simulink model "case1"  (R2024b)
settings: Solver=FixedStepAuto  StartTime=0  StopTime=1  FixedStep=1e-7  RelTol=1e-3
values from neighbouring files (symbols this model uses):
  SG_D_1_D = 0.01056    [IEEE9_case_parameters.m]    (also in case1_parameters.m; case2_parameters.m; case3_parameters.m; case4_parameters.m)
  SG_D_1_EnableSaturation = 0    [IEEE9_case_parameters.m]    (also in case1_parameters.m; case2_parameters.m; case3_parameters.m; case4_parameters.m)
  SG_D_1_f0 = 60    [IEEE9_case_parameters.m]    (also in case1_parameters.m; case2_parameters.m; case3_parameters.m; case4_parameters.m)
  SG_D_1_H = 7.5    [IEEE9_case_parameters.m]    (also in case1_parameters.m; case2_parameters.m; case3_parameters.m; case4_parameters.m)
  SG_D_1_K_A = 20    [IEEE9_case_parameters.m]    (also in case1_parameters.m; case2_parameters.m; case3_parameters.m; case4_parameters.m)
  SG_D_1_K_E = 1.000000e+1    (= 10)    [IEEE9_case_parameters.m]    (also in case1_parameters.m; case2_parameters.m; case3_parameters.m; case4_parameters.m)
  SG_D_1_K_F = 2.363    [IEEE9_case_parameters.m]    (also in case1_parameters.m; case2_parameters.m; case3_parameters.m; case4_parameters.m)
  SG_D_1_K_s = 0.5    [IEEE9_case_parameters.m]    (also in case1_parameters.m = 5; case2_parameters.m = 5; case3_parameters.m = 5; case4_parameters.m = 5)
  SG_D_1_R_a = 0.001088    [IEEE9_case_parameters.m]    (also in case1_parameters.m; case2_parameters.m; case3_parameters.m; case4_parameters.m)
  SG_D_1_S_A = 1    [IEEE9_case_parameters.m]    (also in case1_parameters.m; case2_parameters.m; case3_parameters.m; case4_parameters.m)
  SG_D_1_S_B = 0.103    [IEEE9_case_parameters.m]    (also in case1_parameters.m; case2_parameters.m; case3_parameters.m; case4_parameters.m)
  SG_D_1_S_N = 10.659857    [IEEE9_case_parameters.m]    (also in case1_parameters.m; case2_parameters.m; case3_parameters.m; case4_parameters.m)
  SG_D_1_SpeedPara = 200    [IEEE9_case_parameters.m]    (also in case1_parameters.m; case2_parameters.m; case3_parameters.m; case4_parameters.m)
  SG_D_1_T_0 = 0.720173    [IEEE9_case_parameters.m]    (also in case1_parameters.m = 0.755522; case2_parameters.m = 0.808931; case3_parameters.m = 0.869402; case4_parameters.m = 0.729316)
  SG_D_1_T_1 = 0.3    [IEEE9_case_parameters.m]    (also in case1_parameters.m; case2_parameters.m; case3_parameters.m; case4_parameters.m)
  SG_D_1_T_2 = 0.05    [IEEE9_case_parameters.m]    (also in case1_parameters.m; case2_parameters.m; case3_parameters.m; case4_parameters.m)
  SG_D_1_T_3 = 0.02    [IEEE9_case_parameters.m]    (also in case1_parameters.m; case2_parameters.m; case3_parameters.m; case4_parameters.m)
  SG_D_1_T_4 = 0.005    [IEEE9_case_parameters.m]    (also in case1_parameters.m; case2_parameters.m; case3_parameters.m; case4_parameters.m)
  SG_D_1_T_A = 0.02    [IEEE9_case_parameters.m]    (also in case1_parameters.m; case2_parameters.m; case3_parameters.m; case4_parameters.m)
  SG_D_1_T_dd = 8.000000e+0    (= 8)    [IEEE9_case_parameters.m]    (also in case1_parameters.m; case2_parameters.m; case3_parameters.m; case4_parameters.m)
  SG_D_1_T_ddd = 0.04    [IEEE9_case_parameters.m]    (also in case1_parameters.m; case2_parameters.m; case3_parameters.m; case4_parameters.m)
  SG_D_1_T_E = 0.314    [IEEE9_case_parameters.m]    (also in case1_parameters.m; case2_parameters.m; case3_parameters.m; case4_parameters.m)
  SG_D_1_T_F = 0.35    [IEEE9_case_parameters.m]    (also in case1_parameters.m; case2_parameters.m; case3_parameters.m; case4_parameters.m)
  SG_D_1_T_qd = 0.8    [IEEE9_case_parameters.m]    (also in case1_parameters.m; case2_parameters.m; case3_parameters.m; case4_parameters.m)
  SG_D_1_T_qdd = 0.02    [IEEE9_case_parameters.m]    (also in case1_parameters.m; case2_parameters.m; case3_parameters.m; case4_parameters.m)
  SG_D_1_T_speed = 0.1    [IEEE9_case_parameters.m]    (also in case1_parameters.m = 200; case2_parameters.m = 200; case3_parameters.m = 200; case4_parameters.m = 200)
  SG_D_1_T_w = 0.5    [IEEE9_case_parameters.m]    (also in case1_parameters.m; case2_parameters.m; case3_parameters.m; case4_parameters.m)
  SG_D_1_V_ref = 1.990276    [IEEE9_case_parameters.m]    (also in case1_parameters.m = 2.042296; case2_parameters.m = 2.051388; case3_parameters.m = 2.089584; case4_parameters.m = 2.01845)
  SG_D_1_w_ref = 376.991118    [IEEE9_case_parameters.m]    (also in case1_parameters.m; case2_parameters.m; case3_parameters.m; case4_parameters.m)
  SG_D_1_wb = 6.000000e+1    (= 60)    [IEEE9_case_parameters.m]    (also in case1_parameters.m; case2_parameters.m; case3_parameters.m; case4_parameters.m)
  SG_D_1_x_d = 1.9    [IEEE9_case_parameters.m]    (also in case1_parameters.m; case2_parameters.m; case3_parameters.m; case4_parameters.m)
  SG_D_1_x_dd = 0.302    [IEEE9_case_parameters.m]    (also in case1_parameters.m; case2_parameters.m; case3_parameters.m; case4_parameters.m)
  SG_D_1_x_ddd = 0.204    [IEEE9_case_parameters.m]    (also in case1_parameters.m; case2_parameters.m; case3_parameters.m; case4_parameters.m)
  SG_D_1_x_l = 0.05    [IEEE9_case_parameters.m]    (also in case1_parameters.m; case2_parameters.m; case3_parameters.m; case4_parameters.m)
  SG_D_1_x_q = 1.3    [IEEE9_case_parameters.m]    (also in case1_parameters.m; case2_parameters.m; case3_parameters.m; case4_parameters.m)
  SG_D_1_x_qd = 0.5    [IEEE9_case_parameters.m]    (also in case1_parameters.m; case2_parameters.m; case3_parameters.m; case4_parameters.m)
  SG_D_1_x_qdd = 0.3    [IEEE9_case_parameters.m]    (also in case1_parameters.m; case2_parameters.m; case3_parameters.m; case4_parameters.m)
  SG_D_2_D = 0.02    [IEEE9_case_parameters.m]    (also in case1_parameters.m; case2_parameters.m; case3_parameters.m; case4_parameters.m)
  SG_D_2_EnableSaturation = 0    [IEEE9_case_parameters.m]    (also in case1_parameters.m; case2_parameters.m; case3_parameters.m; case4_parameters.m)
  SG_D_2_f0 = 60    [IEEE9_case_parameters.m]    (also in case1_parameters.m; case2_parameters.m; case3_parameters.m; case4_parameters.m)
  SG_D_2_H = 8.000000e+0    (= 8)    [IEEE9_case_parameters.m]    (also in case1_parameters.m; case2_parameters.m; case3_parameters.m; case4_parameters.m)
  SG_D_2_K_A = 20    [IEEE9_case_parameters.m]    (also in case1_parameters.m; case2_parameters.m; case3_parameters.m; case4_parameters.m)
  SG_D_2_K_E = 1.000000e+1    (= 10)    [IEEE9_case_parameters.m]    (also in case1_parameters.m; case2_parameters.m; case3_parameters.m; case4_parameters.m)
  SG_D_2_K_F = 2.363    [IEEE9_case_parameters.m]    (also in case1_parameters.m; case2_parameters.m; case3_parameters.m; case4_parameters.m)
  SG_D_2_K_s = 0.5    [IEEE9_case_parameters.m]    (also in case1_parameters.m = 4; case2_parameters.m = 4; case3_parameters.m = 4; case4_parameters.m = 4)
  SG_D_2_R_a = 0.001088    [IEEE9_case_parameters.m]    (also in case1_parameters.m; case2_parameters.m; case3_parameters.m; case4_parameters.m)
  SG_D_2_S_A = 1    [IEEE9_case_parameters.m]    (also in case1_parameters.m; case2_parameters.m; case3_parameters.m; case4_parameters.m)
  SG_D_2_S_B = 0.103    [IEEE9_case_parameters.m]    (also in case1_parameters.m; case2_parameters.m; case3_parameters.m; case4_parameters.m)
  SG_D_2_S_N = 10.659857    [IEEE9_case_parameters.m]    (also in case1_parameters.m; case2_parameters.m; case3_parameters.m; case4_parameters.m)
  SG_D_2_SpeedPara = 200    [IEEE9_case_parameters.m]    (also in case1_parameters.m; case2_parameters.m; case3_parameters.m; case4_parameters.m)
  SG_D_2_T_0 = 1.632913    [IEEE9_case_parameters.m]    (also in case1_parameters.m = 1.632925; case2_parameters.m = 1.632915; case3_parameters.m = 1.632914; case4_parameters.m = 1.632927)
  SG_D_2_T_1 = 0.2    [IEEE9_case_parameters.m]    (also in case1_parameters.m; case2_parameters.m; case3_parameters.m; case4_parameters.m)
  SG_D_2_T_2 = 0.05    [IEEE9_case_parameters.m]    (also in case1_parameters.m; case2_parameters.m; case3_parameters.m; case4_parameters.m)
  SG_D_2_T_3 = 0.02    [IEEE9_case_parameters.m]    (also in case1_parameters.m; case2_parameters.m; case3_parameters.m; case4_parameters.m)
  SG_D_2_T_4 = 0.005    [IEEE9_case_parameters.m]    (also in case1_parameters.m; case2_parameters.m; case3_parameters.m; case4_parameters.m)
  SG_D_2_T_A = 0.02    [IEEE9_case_parameters.m]    (also in case1_parameters.m; case2_parameters.m; case3_parameters.m; case4_parameters.m)
  SG_D_2_T_dd = 7.9    [IEEE9_case_parameters.m]    (also in case1_parameters.m; case2_parameters.m; case3_parameters.m; case4_parameters.m)
  SG_D_2_T_ddd = 0.04    [IEEE9_case_parameters.m]    (also in case1_parameters.m; case2_parameters.m; case3_parameters.m; case4_parameters.m)
  SG_D_2_T_E = 0.314    [IEEE9_case_parameters.m]    (also in case1_parameters.m; case2_parameters.m; case3_parameters.m; case4_parameters.m)
  SG_D_2_T_F = 0.35    [IEEE9_case_parameters.m]    (also in case1_parameters.m; case2_parameters.m; case3_parameters.m; case4_parameters.m)
  SG_D_2_T_qd = 0.8    [IEEE9_case_parameters.m]    (also in case1_parameters.m; case2_parameters.m; case3_parameters.m; case4_parameters.m)
  SG_D_2_T_qdd = 0.015    [IEEE9_case_parameters.m]    (also in case1_parameters.m; case2_parameters.m; case3_parameters.m; case4_parameters.m)
  SG_D_2_T_speed = 0.1    [IEEE9_case_parameters.m]    (also in case1_parameters.m = 150; case2_parameters.m = 150; case3_parameters.m = 150; case4_parameters.m = 150)
  SG_D_2_T_w = 0.35    [IEEE9_case_parameters.m]    (also in case1_parameters.m; case2_parameters.m; case3_parameters.m; case4_parameters.m)
  SG_D_2_V_ref = 2.58547    [IEEE9_case_parameters.m]    (also in case1_parameters.m = 2.597896; case2_parameters.m = 2.587136; case3_parameters.m = 2.586042; case4_parameters.m = 2.599679)
  SG_D_2_w_ref = 376.991118    [IEEE9_case_parameters.m]    (also in case1_parameters.m; case2_parameters.m; case3_parameters.m; case4_parameters.m)
  SG_D_2_wb = 6.000000e+1    (= 60)    [IEEE9_case_parameters.m]    (also in case1_parameters.m; case2_parameters.m; case3_parameters.m; case4_parameters.m)
  SG_D_2_x_d = 1.8    [IEEE9_case_parameters.m]    (also in case1_parameters.m; case2_parameters.m; case3_parameters.m; case4_parameters.m)
  SG_D_2_x_dd = 0.302    [IEEE9_case_parameters.m]    (also in case1_parameters.m; case2_parameters.m; case3_parameters.m; case4_parameters.m)
  SG_D_2_x_ddd = 0.204    [IEEE9_case_parameters.m]    (also in case1_parameters.m; case2_parameters.m; case3_parameters.m; case4_parameters.m)
  SG_D_2_x_l = 0.05    [IEEE9_case_parameters.m]    (also in case1_parameters.m; case2_parameters.m; case3_parameters.m; case4_parameters.m)
  SG_D_2_x_q = 1.25    [IEEE9_case_parameters.m]    (also in case1_parameters.m; case2_parameters.m; case3_parameters.m; case4_parameters.m)
  SG_D_2_x_qd = 0.5    [IEEE9_case_parameters.m]    (also in case1_parameters.m; case2_parameters.m; case3_parameters.m; case4_parameters.m)
  SG_D_2_x_qdd = 0.3    [IEEE9_case_parameters.m]    (also in case1_parameters.m; case2_parameters.m; case3_parameters.m; case4_parameters.m)
  SG_D_3_D = 0.02    [IEEE9_case_parameters.m]    (also in case1_parameters.m; case2_parameters.m; case3_parameters.m; case4_parameters.m)
  SG_D_3_EnableSaturation = 0    [IEEE9_case_parameters.m]    (also in case1_parameters.m; case2_parameters.m; case3_parameters.m; case4_parameters.m)
  SG_D_3_f0 = 60    [IEEE9_case_parameters.m]    (also in case1_parameters.m; case2_parameters.m; case3_parameters.m; case4_parameters.m)
  SG_D_3_H = 7.7    [IEEE9_case_parameters.m]    (also in case1_parameters.m; case2_parameters.m; case3_parameters.m; case4_parameters.m)
  SG_D_3_K_A = 20    [IEEE9_case_parameters.m]    (also in case1_parameters.m; case2_parameters.m; case3_parameters.m; case4_parameters.m)
  SG_D_3_K_E = 1.000000e+1    (= 10)    [IEEE9_case_parameters.m]    (also in case1_parameters.m; case2_parameters.m; case3_parameters.m; case4_parameters.m)
  SG_D_3_K_F = 2.363    [IEEE9_case_parameters.m]    (also in case1_parameters.m; case2_parameters.m; case3_parameters.m; case4_parameters.m)
  SG_D_3_K_s = 0.2    [IEEE9_case_parameters.m]    (also in case1_parameters.m = 2; case2_parameters.m = 2; case3_parameters.m = 2; case4_parameters.m = 2)
  SG_D_3_R_a = 0.001088    [IEEE9_case_parameters.m]    (also in case1_parameters.m; case2_parameters.m; case3_parameters.m; case4_parameters.m)
  SG_D_3_S_A = 1    [IEEE9_case_parameters.m]    (also in case1_parameters.m; case2_parameters.m; case3_parameters.m; case4_parameters.m)
  SG_D_3_S_B = 0.103    [IEEE9_case_parameters.m]    (also in case1_parameters.m; case2_parameters.m; case3_parameters.m; case4_parameters.m)
  SG_D_3_S_N = 10.659857    [IEEE9_case_parameters.m]    (also in case1_parameters.m; case2_parameters.m; case3_parameters.m; case4_parameters.m)
  SG_D_3_SpeedPara = 200    [IEEE9_case_parameters.m]    (also in case1_parameters.m; case2_parameters.m; case3_parameters.m; case4_parameters.m)
  SG_D_3_T_0 = 0.850788    [IEEE9_case_parameters.m]    (also in case1_parameters.m = 0.850786; case2_parameters.m = 0.850787; case3_parameters.m; case4_parameters.m = 0.850786)
  SG_D_3_T_1 = 0.2    [IEEE9_case_parameters.m]    (also in case1_parameters.m; case2_parameters.m; case3_parameters.m; case4_parameters.m)
  SG_D_3_T_2 = 0.05    [IEEE9_case_parameters.m]    (also in case1_parameters.m; case2_parameters.m; case3_parameters.m; case4_parameters.m)
  SG_D_3_T_3 = 0.02    [IEEE9_case_parameters.m]    (also in case1_parameters.m; case2_parameters.m; case3_parameters.m; case4_parameters.m)
  SG_D_3_T_4 = 0.005    [IEEE9_case_parameters.m]    (also in case1_parameters.m; case2_parameters.m; case3_parameters.m; case4_parameters.m)
  SG_D_3_T_A = 0.02    [IEEE9_case_parameters.m]    (also in case1_parameters.m; case2_parameters.m; case3_parameters.m; case4_parameters.m)
  SG_D_3_T_dd = 8.1    [IEEE9_case_parameters.m]    (also in case1_parameters.m; case2_parameters.m; case3_parameters.m; case4_parameters.m)
  SG_D_3_T_ddd = 0.04    [IEEE9_case_parameters.m]    (also in case1_parameters.m; case2_parameters.m; case3_parameters.m; case4_parameters.m)
  SG_D_3_T_E = 0.314    [IEEE9_case_parameters.m]    (also in case1_parameters.m; case2_parameters.m; case3_parameters.m; case4_parameters.m)
  SG_D_3_T_F = 0.35    [IEEE9_case_parameters.m]    (also in case1_parameters.m; case2_parameters.m; case3_parameters.m; case4_parameters.m)
  SG_D_3_T_qd = 0.8    [IEEE9_case_parameters.m]    (also in case1_parameters.m; case2_parameters.m; case3_parameters.m; case4_parameters.m)
  SG_D_3_T_qdd = 0.015    [IEEE9_case_parameters.m]    (also in case1_parameters.m; case2_parameters.m; case3_parameters.m; case4_parameters.m)
  SG_D_3_T_speed = 0.1    [IEEE9_case_parameters.m]    (also in case1_parameters.m = 180; case2_parameters.m = 180; case3_parameters.m = 180; case4_parameters.m = 180)
  SG_D_3_T_w = 0.4    [IEEE9_case_parameters.m]    (also in case1_parameters.m; case2_parameters.m; case3_parameters.m; case4_parameters.m)
  SG_D_3_V_ref = 1.892727    [IEEE9_case_parameters.m]    (also in case1_parameters.m = 1.906439; case2_parameters.m = 1.895535; case3_parameters.m = 1.892105; case4_parameters.m = 1.906598)
  SG_D_3_w_ref = 376.991118    [IEEE9_case_parameters.m]    (also in case1_parameters.m; case2_parameters.m; case3_parameters.m; case4_parameters.m)
  SG_D_3_wb = 6.000000e+1    (= 60)    [IEEE9_case_parameters.m]    (also in case1_parameters.m; case2_parameters.m; case3_parameters.m; case4_parameters.m)
  SG_D_3_x_d = 1.85    [IEEE9_case_parameters.m]    (also in case1_parameters.m; case2_parameters.m; case3_parameters.m; case4_parameters.m)
  SG_D_3_x_dd = 0.302    [IEEE9_case_parameters.m]    (also in case1_parameters.m; case2_parameters.m; case3_parameters.m; case4_parameters.m)
  SG_D_3_x_ddd = 0.204    [IEEE9_case_parameters.m]    (also in case1_parameters.m; case2_parameters.m; case3_parameters.m; case4_parameters.m)
  SG_D_3_x_l = 0.05    [IEEE9_case_parameters.m]    (also in case1_parameters.m; case2_parameters.m; case3_parameters.m; case4_parameters.m)
  SG_D_3_x_q = 1.2    [IEEE9_case_parameters.m]    (also in case1_parameters.m; case2_parameters.m; case3_parameters.m; case4_parameters.m)
  SG_D_3_x_qd = 0.5    [IEEE9_case_parameters.m]    (also in case1_parameters.m; case2_parameters.m; case3_parameters.m; case4_parameters.m)
  SG_D_3_x_qdd = 0.3    [IEEE9_case_parameters.m]    (also in case1_parameters.m; case2_parameters.m; case3_parameters.m; case4_parameters.m)
(part 3 of 12)

== system case1/AC_1/d_id_load_7_block ==
  note: d_id_load_7 in case1
      | $376.991118430775\,\mathrm{iq}_{\mathrm{load},7}-1025.52197474754\,\mathrm{id}_{\mathrm{load},7}+1219.07936641917\,\mathrm{vd}_{\mathrm{bus},7}$
      | Automatically generated on 2025-10-31 18:50:38 .
  State_id_load_7_7e244 : Inport
  State_iq_load_7_7baed : Inport  Port=2
  State_vd_bus_7_6ff07 : Inport  Port=3
  Add_61909 : Sum
  Add_b6594 : Sum
  Constant_-1025.52197474754_80390 : Constant  Value=-1025.52197474754
  Constant_1219.07936641917_674e5 : Constant  Value=1219.07936641917
  Constant_376.991118430775_4e2b0 : Constant  Value=376.991118430775
  Product_12f11 : Product
  Product_491b3 : Product
  Product_d0252 : Product
  Blockout_d_id_load_7_3ab02 : Outport
  wires:
  Constant_-1025.52197474754_80390/1 -> Product_12f11/1
  Product_491b3/1 -> Add_b6594/2
  State_id_load_7_7e244/1 -> Product_12f11/2
  Constant_376.991118430775_4e2b0/1 -> Product_491b3/1
  Product_12f11/1 -> Add_b6594/1
  State_iq_load_7_7baed/1 -> Product_491b3/2
  Constant_1219.07936641917_674e5/1 -> Product_d0252/1
  State_vd_bus_7_6ff07/1 -> Product_d0252/2
  Add_b6594/1 -> Add_61909/1
  Product_d0252/1 -> Add_61909/2
  Add_61909/1 -> Blockout_d_id_load_7_3ab02/1

== system case1/AC_1/d_id_load_9_block ==
  note: d_id_load_9 in case1
      | $376.991118430775\,\mathrm{iq}_{\mathrm{load},9}-897.331727994337\,\mathrm{id}_{\mathrm{load},9}+1471.75490379155\,\mathrm{vd}_{\mathrm{bus},9}$
      | Automatically generated on 2025-10-31 18:50:40 .
  State_id_load_9_6175e : Inport
  State_iq_load_9_2b565 : Inport  Port=2
  State_vd_bus_9_97729 : Inport  Port=3
  Add_41749 : Sum
  Add_a1c56 : Sum
  Constant_-897.331727994337_48efa : Constant  Value=-897.331727994337
  Constant_1471.75490379155_76577 : Constant  Value=1471.75490379155
  Constant_376.991118430775_bbee5 : Constant  Value=376.991118430775
  Product_0f7c0 : Product
  Product_ef85c : Product
  Product_fef82 : Product
  Blockout_d_id_load_9_6afbf : Outport
  wires:
  Constant_-897.331727994337_48efa/1 -> Product_0f7c0/1
  Product_fef82/1 -> Add_a1c56/2
  State_id_load_9_6175e/1 -> Product_0f7c0/2
  Constant_376.991118430775_bbee5/1 -> Product_fef82/1
  Product_0f7c0/1 -> Add_a1c56/1
  State_iq_load_9_2b565/1 -> Product_fef82/2
  Constant_1471.75490379155_76577/1 -> Product_ef85c/1
  State_vd_bus_9_97729/1 -> Product_ef85c/2
  Add_a1c56/1 -> Add_41749/1
  Product_ef85c/1 -> Add_41749/2
  Add_41749/1 -> Blockout_d_id_load_9_6afbf/1

== system case1/AC_1/d_iq_line_1_4_block ==
  note: d_iq_line_1_4 in case1
      | $6387.9543042679\,\mathrm{vq}_{\mathrm{bus},1}-376.991118430775\,\mathrm{id}_{\mathrm{line},1,4}-6387.9543042679\,\mathrm{vq}_{\mathrm{bus},4}$
      | Automatically generated on 2025-10-31 18:50:43 .
  State_id_line_1_4_e2784 : Inport
  State_vq_bus_1_cc1a1 : Inport  Port=2
  State_vq_bus_4_b95c1 : Inport  Port=3
  Add_609df : Sum
  Constant_-376.991118430775_4f7c2 : Constant  Value=-376.991118430775
  Constant_6387.9543042679_077c5 : Constant  Value=6387.9543042679
  Constant_6387.9543042679_526d1 : Constant  Value=6387.9543042679
  Product_10305 : Product
  Product_2fb22 : Product
  Product_4450d : Product
  Subtract_016be : Sum  Inputs=+-
  Blockout_d_iq_line_1_4_78aac : Outport
  wires:
  Constant_-376.991118430775_4f7c2/1 -> Product_10305/1
  Product_2fb22/1 -> Add_609df/2
  State_id_line_1_4_e2784/1 -> Product_10305/2
  Constant_6387.9543042679_526d1/1 -> Product_2fb22/1
  Product_10305/1 -> Add_609df/1
  Subtract_016be/1 -> Blockout_d_iq_line_1_4_78aac/1
  State_vq_bus_1_cc1a1/1 -> Product_2fb22/2
  Constant_6387.9543042679_077c5/1 -> Product_4450d/1
  State_vq_bus_4_b95c1/1 -> Product_4450d/2
  Add_609df/1 -> Subtract_016be/1
  Product_4450d/1 -> Subtract_016be/2

== system case1/AC_1/d_iq_line_3_6_block ==
  note: d_iq_line_3_6 in case1
      | $6278.9448451507\,\mathrm{vq}_{\mathrm{bus},3}-376.991118430775\,\mathrm{id}_{\mathrm{line},3,6}-6278.9448451507\,\mathrm{vq}_{\mathrm{bus},6}$
      | Automatically generated on 2025-10-31 18:50:50 .
  State_id_line_3_6_f913b : Inport
  State_vq_bus_3_5a1c9 : Inport  Port=2
  State_vq_bus_6_03933 : Inport  Port=3
  Add_de142 : Sum
  Constant_-376.991118430775_59102 : Constant  Value=-376.991118430775
  Constant_6278.9448451507_1221b : Constant  Value=6278.9448451507
  Constant_6278.9448451507_5b025 : Constant  Value=6278.9448451507
  Product_669f2 : Product
  Product_75886 : Product
  Product_e6f36 : Product
  Subtract_db1d0 : Sum  Inputs=+-
  Blockout_d_iq_line_3_6_784c0 : Outport
  wires:
  Constant_-376.991118430775_59102/1 -> Product_75886/1
  Product_e6f36/1 -> Add_de142/2
  State_id_line_3_6_f913b/1 -> Product_75886/2
  Constant_6278.9448451507_1221b/1 -> Product_e6f36/1
  Product_75886/1 -> Add_de142/1
  State_vq_bus_3_5a1c9/1 -> Product_e6f36/2
  Constant_6278.9448451507_5b025/1 -> Product_669f2/1
  State_vq_bus_6_03933/1 -> Product_669f2/2
  Add_de142/1 -> Subtract_db1d0/1
  Product_669f2/1 -> Subtract_db1d0/2
  Subtract_db1d0/1 -> Blockout_d_iq_line_3_6_784c0/1

== system case1/AC_1/d_iq_line_4_5_block ==
  note: d_iq_line_4_5 in case1
      | $3999.41486875903\,\mathrm{vq}_{\mathrm{bus},4}-70.7030565753656\,\mathrm{iq}_{\mathrm{line},4,5}-376.991118430775\,\mathrm{id}_{\mathrm{line},4,5}-3999.41486875903\,\mathrm{vq}_{\mathrm{bus},5}$
      | Automatically generated on 2025-10-31 18:50:45 .
  State_id_line_4_5_305b5 : Inport
  State_iq_line_4_5_0a9d2 : Inport  Port=2
  State_vq_bus_4_e89f1 : Inport  Port=3
  State_vq_bus_5_04a69 : Inport  Port=4
  Add_d0e3e : Sum
  Constant_-376.991118430775_c3725 : Constant  Value=-376.991118430775
  Constant_3999.41486875903_a8499 : Constant  Value=3999.41486875903
  Constant_3999.41486875903_f6b00 : Constant  Value=3999.41486875903
  Constant_70.7030565753656_055d7 : Constant  Value=70.7030565753656
  Product_4f6ce : Product
  Product_504af : Product
  Product_52caf : Product
  Product_aa46e : Product
  Subtract_8fbf3 : Sum  Inputs=+-
  Subtract_f2a4b : Sum  Inputs=+-
  Blockout_d_iq_line_4_5_e1e40 : Outport
  wires:
  Constant_-376.991118430775_c3725/1 -> Product_504af/1
  Constant_70.7030565753656_055d7/1 -> Product_aa46e/1
  State_id_line_4_5_305b5/1 -> Product_504af/2
  State_iq_line_4_5_0a9d2/1 -> Product_aa46e/2
  Product_504af/1 -> Subtract_8fbf3/1
  Constant_3999.41486875903_a8499/1 -> Product_52caf/1
  Product_aa46e/1 -> Subtract_8fbf3/2
  State_vq_bus_4_e89f1/1 -> Product_52caf/2
  Subtract_8fbf3/1 -> Add_d0e3e/1
  Product_52caf/1 -> Add_d0e3e/2
  Constant_3999.41486875903_f6b00/1 -> Product_4f6ce/1
  State_vq_bus_5_04a69/1 -> Product_4f6ce/2
  Add_d0e3e/1 -> Subtract_f2a4b/1
  Product_4f6ce/1 -> Subtract_f2a4b/2
  Subtract_f2a4b/1 -> Blockout_d_iq_line_4_5_e1e40/1

== system case1/AC_1/d_iq_line_5_6_block ==
  note: d_iq_line_5_6 in case1
      | $2164.38922309312\,\mathrm{vq}_{\mathrm{bus},5}-87.7794349454712\,\mathrm{iq}_{\mathrm{line},5,6}-376.991118430775\,\mathrm{id}_{\mathrm{line},5,6}-2164.38922309312\,\mathrm{vq}_{\mathrm{bus},6}$
      | Automatically generated on 2025-10-31 18:50:48 .
  State_id_line_5_6_4698d : Inport
  State_iq_line_5_6_e5c27 : Inport  Port=2
  State_vq_bus_5_b22ab : Inport  Port=3
  State_vq_bus_6_bf656 : Inport  Port=4
  Add_a83be : Sum
  Constant_-376.991118430775_4d48f : Constant  Value=-376.991118430775
  Constant_2164.38922309312_70a07 : Constant  Value=2164.38922309312
  Constant_2164.38922309312_f6087 : Constant  Value=2164.38922309312
  Constant_87.7794349454712_08c9f : Constant  Value=87.7794349454712
  Product_0ca73 : Product
  Product_18bd1 : Product
  Product_3d32a : Product
  Product_b60ba : Product
  Subtract_1282d : Sum  Inputs=+-
  Subtract_42846 : Sum  Inputs=+-
  Blockout_d_iq_line_5_6_8d1bb : Outport
  wires:
  Constant_-376.991118430775_4d48f/1 -> Product_3d32a/1
  Constant_87.7794349454712_08c9f/1 -> Product_0ca73/1
  Subtract_1282d/1 -> Blockout_d_iq_line_5_6_8d1bb/1
  State_id_line_5_6_4698d/1 -> Product_3d32a/2
  State_iq_line_5_6_e5c27/1 -> Product_0ca73/2
  Product_3d32a/1 -> Subtract_42846/1
  Constant_2164.38922309312_f6087/1 -> Product_b60ba/1
  Product_0ca73/1 -> Subtract_42846/2
  Product_18bd1/1 -> Subtract_1282d/2
  State_vq_bus_5_b22ab/1 -> Product_b60ba/2
  Subtract_42846/1 -> Add_a83be/1
  Product_b60ba/1 -> Add_a83be/2
  Constant_2164.38922309312_70a07/1 -> Product_18bd1/1
  State_vq_bus_6_bf656/1 -> Product_18bd1/2
  Add_a83be/1 -> Subtract_1282d/1

== system case1/AC_1/d_iq_line_6_7_block ==
  note: d_iq_line_6_7 in case1
      | $3650.2596024388\,\mathrm{vq}_{\mathrm{bus},6}-45.1713972564836\,\mathrm{iq}_{\mathrm{line},6,7}-376.991118430775\,\mathrm{id}_{\mathrm{line},6,7}-3650.2596024388\,\mathrm{vq}_{\mathrm{bus},7}$
      | Automatically generated on 2025-10-31 18:50:52 .
  State_id_line_6_7_d6333 : Inport
  State_iq_line_6_7_6494b : Inport  Port=2
  State_vq_bus_6_af623 : Inport  Port=3
  State_vq_bus_7_386f3 : Inport  Port=4
  Add_1f3e0 : Sum
  Constant_-376.991118430775_f3922 : Constant  Value=-376.991118430775
  Constant_3650.2596024388_32c77 : Constant  Value=3650.2596024388
  Constant_3650.2596024388_bb62a : Constant  Value=3650.2596024388
  Constant_45.1713972564836_4ebf7 : Constant  Value=45.1713972564836
  Product_58448 : Product
  Product_5c0e6 : Product
  Product_7400f : Product
  Product_cdcfd : Product
  Subtract_13a48 : Sum  Inputs=+-
  Subtract_ef767 : Sum  Inputs=+-
  Blockout_d_iq_line_6_7_6cbac : Outport
  wires:
  Constant_-376.991118430775_f3922/1 -> Product_cdcfd/1
  Constant_45.1713972564836_4ebf7/1 -> Product_7400f/1
  State_id_line_6_7_d6333/1 -> Product_cdcfd/2
  State_iq_line_6_7_6494b/1 -> Product_7400f/2
  Product_cdcfd/1 -> Subtract_ef767/1
  Constant_3650.2596024388_32c77/1 -> Product_58448/1
  Product_7400f/1 -> Subtract_ef767/2
  State_vq_bus_6_af623/1 -> Product_58448/2
  Subtract_ef767/1 -> Add_1f3e0/1
  Product_58448/1 -> Add_1f3e0/2
  Constant_3650.2596024388_bb62a/1 -> Product_5c0e6/1
  State_vq_bus_7_386f3/1 -> Product_5c0e6/2
  Add_1f3e0/1 -> Subtract_13a48/1
  Product_5c0e6/1 -> Subtract_13a48/2
  Subtract_13a48/1 -> Blockout_d_iq_line_6_7_6cbac/1

== system case1/AC_1/d_iq_line_7_8_block ==
  note: d_iq_line_7_8 in case1
      | $5110.36344341432\,\mathrm{vq}_{\mathrm{bus},7}-45.1713972564836\,\mathrm{iq}_{\mathrm{line},7,8}-376.991118430775\,\mathrm{id}_{\mathrm{line},7,8}-5110.36344341432\,\mathrm{vq}_{\mathrm{bus},8}$
      | Automatically generated on 2025-10-31 18:50:55 .
  State_id_line_7_8_27216 : Inport
  State_iq_line_7_8_50859 : Inport  Port=2
  State_vq_bus_7_1c43c : Inport  Port=3
  State_vq_bus_8_5c564 : Inport  Port=4
  Add_9974c : Sum
  Constant_-376.991118430775_c1de4 : Constant  Value=-376.991118430775
  Constant_45.1713972564836_434ff : Constant  Value=45.1713972564836
  Constant_5110.36344341432_15b95 : Constant  Value=5110.36344341432
  Constant_5110.36344341432_a2de5 : Constant  Value=5110.36344341432
  Product_4df6e : Product
  Product_76d6a : Product
  Product_92a22 : Product
  Product_e4bcb : Product
  Subtract_af39e : Sum  Inputs=+-
  Subtract_f0d3e : Sum  Inputs=+-
  Blockout_d_iq_line_7_8_28933 : Outport
  wires:
  Constant_-376.991118430775_c1de4/1 -> Product_92a22/1
  Constant_45.1713972564836_434ff/1 -> Product_4df6e/1
  State_id_line_7_8_27216/1 -> Product_92a22/2
  State_iq_line_7_8_50859/1 -> Product_4df6e/2
  Product_92a22/1 -> Subtract_f0d3e/1
  Constant_5110.36344341432_a2de5/1 -> Product_e4bcb/1
  Product_4df6e/1 -> Subtract_f0d3e/2
  State_vq_bus_7_1c43c/1 -> Product_e4bcb/2
  Subtract_f0d3e/1 -> Add_9974c/1
  Product_e4bcb/1 -> Add_9974c/2
  Constant_5110.36344341432_15b95/1 -> Product_76d6a/1
  State_vq_bus_8_5c564/1 -> Product_76d6a/2
  Add_9974c/1 -> Subtract_af39e/1
  Product_76d6a/1 -> Subtract_af39e/2
  Subtract_af39e/1 -> Blockout_d_iq_line_7_8_28933/1

== system case1/AC_1/d_iq_line_8_2_block ==
  note: d_iq_line_8_2 in case1
      | $5887.13868681329\,\mathrm{vq}_{\mathrm{bus},8}-5887.13868681329\,\mathrm{vq}_{\mathrm{bus},2}-376.991118430775\,\mathrm{id}_{\mathrm{line},8,2}$
      | Automatically generated on 2025-10-31 18:50:57 .
  State_id_line_8_2_17219 : Inport
  State_vq_bus_2_eedb1 : Inport  Port=2
  State_vq_bus_8_e41a9 : Inport  Port=3
  Add_3f7c5 : Sum
  Constant_-376.991118430775_236ed : Constant  Value=-376.991118430775
  Constant_5887.13868681329_2f519 : Constant  Value=5887.13868681329
  Constant_5887.13868681329_c624f : Constant  Value=5887.13868681329
  Product_00e9a : Product
  Product_3f111 : Product
  Product_7bb5b : Product
  Subtract_4486f : Sum  Inputs=+-
  Blockout_d_iq_line_8_2_543a1 : Outport
  wires:
  Constant_-376.991118430775_236ed/1 -> Product_7bb5b/1
  Product_3f111/1 -> Subtract_4486f/2
  State_id_line_8_2_17219/1 -> Product_7bb5b/2
  Constant_5887.13868681329_2f519/1 -> Product_3f111/1
  Product_7bb5b/1 -> Subtract_4486f/1
  State_vq_bus_2_eedb1/1 -> Product_3f111/2
  Constant_5887.13868681329_c624f/1 -> Product_00e9a/1
  State_vq_bus_8_e41a9/1 -> Product_00e9a/2
  Subtract_4486f/1 -> Add_3f7c5/1
  Product_00e9a/1 -> Add_3f7c5/2
  Add_3f7c5/1 -> Blockout_d_iq_line_8_2_543a1/1

== system case1/AC_1/d_iq_line_8_9_block ==
  note: d_iq_line_8_9 in case1
      | $2285.37992500516\,\mathrm{vq}_{\mathrm{bus},8}-76.0503465684605\,\mathrm{iq}_{\mathrm{line},8,9}-376.991118430775\,\mathrm{id}_{\mathrm{line},8,9}-2285.37992500516\,\mathrm{vq}_{\mathrm{bus},9}$
      | Automatically generated on 2025-10-31 18:50:59 .
  State_id_line_8_9_64212 : Inport
  State_iq_line_8_9_91aab : Inport  Port=2
  State_vq_bus_8_6b472 : Inport  Port=3
  State_vq_bus_9_3314f : Inport  Port=4
  Add_a4af0 : Sum
  Constant_-376.991118430775_86ed7 : Constant  Value=-376.991118430775
  Constant_2285.37992500516_07c92 : Constant  Value=2285.37992500516
  Constant_2285.37992500516_d49b9 : Constant  Value=2285.37992500516
  Constant_76.0503465684605_525d0 : Constant  Value=76.0503465684605
  Product_6704b : Product
  Product_7b1ff : Product
  Product_a999f : Product
  Product_ba037 : Product
  Subtract_28ea0 : Sum  Inputs=+-
  Subtract_48212 : Sum  Inputs=+-
  Blockout_d_iq_line_8_9_f1949 : Outport
  wires:
  Constant_-376.991118430775_86ed7/1 -> Product_a999f/1
  Constant_76.0503465684605_525d0/1 -> Product_6704b/1
  State_id_line_8_9_64212/1 -> Product_a999f/2
  State_iq_line_8_9_91aab/1 -> Product_6704b/2
  Product_a999f/1 -> Subtract_28ea0/1
  Constant_2285.37992500516_07c92/1 -> Product_7b1ff/1
  Product_6704b/1 -> Subtract_28ea0/2
  State_vq_bus_8_6b472/1 -> Product_7b1ff/2
  Subtract_28ea0/1 -> Add_a4af0/1
  Product_7b1ff/1 -> Add_a4af0/2
  Constant_2285.37992500516_d49b9/1 -> Product_ba037/1
  Add_a4af0/1 -> Subtract_48212/1
  State_vq_bus_9_3314f/1 -> Product_ba037/2
  Product_ba037/1 -> Subtract_48212/2
  Subtract_48212/1 -> Blockout_d_iq_line_8_9_f1949/1

== system case1/AC_1/d_iq_line_9_4_block ==
  note: d_iq_line_9_4 in case1
      | $4328.77844618625\,\mathrm{vq}_{\mathrm{bus},9}-45.0150948438314\,\mathrm{iq}_{\mathrm{line},9,4}-4328.77844618625\,\mathrm{vq}_{\mathrm{bus},4}-376.991118430775\,\mathrm{id}_{\mathrm{line},9,4}$
      | Automatically generated on 2025-10-31 18:51:02 .
  State_id_line_9_4_c7272 : Inport
  State_iq_line_9_4_4bacc : Inport  Port=2
  State_vq_bus_4_fd03e : Inport  Port=3
  State_vq_bus_9_f6455 : Inport  Port=4
  Add_ee4e4 : Sum
  Constant_-376.991118430775_908fa : Constant  Value=-376.991118430775
  Constant_4328.77844618625_568ab : Constant  Value=4328.77844618625
  Constant_4328.77844618625_c597d : Constant  Value=4328.77844618625
  Constant_45.0150948438314_102c5 : Constant  Value=45.0150948438314
  Product_1f97c : Product
  Product_60d75 : Product
  Product_84ecf : Product
  Product_a507a : Product
  Subtract_10b54 : Sum  Inputs=+-
  Subtract_1ba85 : Sum  Inputs=+-
  Blockout_d_iq_line_9_4_f2aeb : Outport
  wires:
  Constant_-376.991118430775_908fa/1 -> Product_84ecf/1
  Constant_45.0150948438314_102c5/1 -> Product_60d75/1
  State_id_line_9_4_c7272/1 -> Product_84ecf/2
  State_iq_line_9_4_4bacc/1 -> Product_60d75/2
  Product_84ecf/1 -> Subtract_10b54/1
  Constant_4328.77844618625_568ab/1 -> Product_a507a/1
  Product_60d75/1 -> Subtract_10b54/2
  State_vq_bus_4_fd03e/1 -> Product_a507a/2
  Subtract_10b54/1 -> Subtract_1ba85/1
  Product_a507a/1 -> Subtract_1ba85/2
  Constant_4328.77844618625_c597d/1 -> Product_1f97c/1
  Add_ee4e4/1 -> Blockout_d_iq_line_9_4_f2aeb/1
  State_vq_bus_9_f6455/1 -> Product_1f97c/2
  Subtract_1ba85/1 -> Add_ee4e4/1
  Product_1f97c/1 -> Add_ee4e4/2

== system case1/AC_1/d_iq_load_5_block ==
  note: d_iq_load_5 in case1
      | $1165.56205079599\,\mathrm{vq}_{\mathrm{bus},5}-1076.79807376298\,\mathrm{iq}_{\mathrm{load},5}-376.991118430775\,\mathrm{id}_{\mathrm{load},5}$
      | Automatically generated on 2025-10-31 18:50:37 .
  State_id_load_5_781f5 : Inport
  State_iq_load_5_1b8dc : Inport  Port=2
  State_vq_bus_5_2f3a6 : Inport  Port=3
  Add_5bfdf : Sum
  Constant_-376.991118430775_f8cd1 : Constant  Value=-376.991118430775
  Constant_1076.79807376298_786a3 : Constant  Value=1076.79807376298
  Constant_1165.56205079599_3ad9c : Constant  Value=1165.56205079599
  Product_3e941 : Product
  Product_8bb05 : Product
  Product_e7f6f : Product
  Subtract_20152 : Sum  Inputs=+-
  Blockout_d_iq_load_5_d2ff1 : Outport
  wires:
  Constant_-376.991118430775_f8cd1/1 -> Product_3e941/1
  Product_8bb05/1 -> Subtract_20152/2
  State_id_load_5_781f5/1 -> Product_3e941/2
  Constant_1076.79807376298_786a3/1 -> Product_8bb05/1
  Product_3e941/1 -> Subtract_20152/1
  State_iq_load_5_1b8dc/1 -> Product_8bb05/2
  Constant_1165.56205079599_3ad9c/1 -> Product_e7f6f/1
  State_vq_bus_5_2f3a6/1 -> Product_e7f6f/2
  Subtract_20152/1 -> Add_5bfdf/1
  Product_e7f6f/1 -> Add_5bfdf/2
  Add_5bfdf/1 -> Blockout_d_iq_load_5_d2ff1/1

== system case1/AC_1/d_iq_load_7_block ==
  note: d_iq_load_7 in case1
      | $1219.07936641917\,\mathrm{vq}_{\mathrm{bus},7}-1025.52197474754\,\mathrm{iq}_{\mathrm{load},7}-376.991118430775\,\mathrm{id}_{\mathrm{load},7}$
      | Automatically generated on 2025-10-31 18:50:39 .
  State_id_load_7_47db6 : Inport
  State_iq_load_7_f715f : Inport  Port=2
  State_vq_bus_7_c9f78 : Inport  Port=3
  Add_0d47b : Sum
  Constant_-376.991118430775_5a8ca : Constant  Value=-376.991118430775
  Constant_1025.52197474754_bc6a4 : Constant  Value=1025.52197474754
  Constant_1219.07936641917_83e6d : Constant  Value=1219.07936641917
  Product_08d18 : Product
  Product_66909 : Product
  Product_7d335 : Product
  Subtract_2e6ac : Sum  Inputs=+-
  Blockout_d_iq_load_7_2f8c2 : Outport
  wires:
  Constant_-376.991118430775_5a8ca/1 -> Product_7d335/1
  Product_66909/1 -> Subtract_2e6ac/2
  State_id_load_7_47db6/1 -> Product_7d335/2
  Constant_1025.52197474754_bc6a4/1 -> Product_66909/1
  Product_7d335/1 -> Subtract_2e6ac/1
  State_iq_load_7_f715f/1 -> Product_66909/2
  Constant_1219.07936641917_83e6d/1 -> Product_08d18/1
  State_vq_bus_7_c9f78/1 -> Product_08d18/2
  Subtract_2e6ac/1 -> Add_0d47b/1
  Product_08d18/1 -> Add_0d47b/2
  Add_0d47b/1 -> Blockout_d_iq_load_7_2f8c2/1

== system case1/AC_1/d_iq_load_9_block ==
  note: d_iq_load_9 in case1
      | $1471.75490379155\,\mathrm{vq}_{\mathrm{bus},9}-897.331727994337\,\mathrm{iq}_{\mathrm{load},9}-376.991118430775\,\mathrm{id}_{\mathrm{load},9}$
      | Automatically generated on 2025-10-31 18:50:41 .
  State_id_load_9_ebd3b : Inport
  State_iq_load_9_2bff1 : Inport  Port=2
  State_vq_bus_9_8e131 : Inport  Port=3
  Add_1cb63 : Sum
  Constant_-376.991118430775_25a42 : Constant  Value=-376.991118430775
  Constant_1471.75490379155_f807b : Constant  Value=1471.75490379155
  Constant_897.331727994337_fd528 : Constant  Value=897.331727994337
  Product_2f195 : Product
  Product_2f2d0 : Product
  Product_5dfae : Product
  Subtract_ccdde : Sum  Inputs=+-
  Blockout_d_iq_load_9_225bd : Outport
  wires:
  Constant_-376.991118430775_25a42/1 -> Product_2f195/1
  Product_5dfae/1 -> Subtract_ccdde/2
  State_id_load_9_ebd3b/1 -> Product_2f195/2
  Add_1cb63/1 -> Blockout_d_iq_load_9_225bd/1
  Constant_897.331727994337_fd528/1 -> Product_5dfae/1
  Product_2f2d0/1 -> Add_1cb63/2
  Product_2f195/1 -> Subtract_ccdde/1
  State_iq_load_9_2bff1/1 -> Product_5dfae/2
  Constant_1471.75490379155_f807b/1 -> Product_2f2d0/1
  State_vq_bus_9_8e131/1 -> Product_2f2d0/2
  Subtract_ccdde/1 -> Add_1cb63/1

== system case1/AC_1/d_vd_bus_1_block ==
  note: d_vd_bus_1 in case1
      | $37699111.8430775\,\mathrm{id}_{\mathrm{bus},1}+376.991118430775\,\mathrm{vq}_{\mathrm{bus},1}$
      | Automatically generated on 2025-10-31 18:50:21 .
  Alge_id_bus_1_738e1 : Inport
  State_vq_bus_1_68a3e : Inport  Port=2
  Add_b9764 : Sum
  Constant_376.991118430775_2a7de : Constant  Value=376.991118430775
  Constant_37699111.8430775_36455 : Constant  Value=37699111.8430775
  Product_7fac8 : Product
  Product_e8551 : Product
  Blockout_d_vd_bus_1_e1401 : Outport
  wires:
  Constant_37699111.8430775_36455/1 -> Product_e8551/1
  Product_7fac8/1 -> Add_b9764/2
  Alge_id_bus_1_738e1/1 -> Product_e8551/2
  Constant_376.991118430775_2a7de/1 -> Product_7fac8/1
  State_vq_bus_1_68a3e/1 -> Product_7fac8/2
  Add_b9764/1 -> Blockout_d_vd_bus_1_e1401/1
  Product_e8551/1 -> Add_b9764/1

== system case1/AC_1/d_vd_bus_2_block ==
  note: d_vd_bus_2 in case1
      | $37699111.8430775\,\mathrm{id}_{\mathrm{bus},2}+376.991118430775\,\mathrm{vq}_{\mathrm{bus},2}$
      | Automatically generated on 2025-10-31 18:50:22 .
  Alge_id_bus_2_38876 : Inport
  State_vq_bus_2_b534c : Inport  Port=2
  Add_7ba88 : Sum
  Constant_376.991118430775_c52dd : Constant  Value=376.991118430775
  Constant_37699111.8430775_e863f : Constant  Value=37699111.8430775
  Product_2bf68 : Product
  Product_2d9be : Product
  Blockout_d_vd_bus_2_81105 : Outport
  wires:
  Constant_37699111.8430775_e863f/1 -> Product_2d9be/1
  Product_2bf68/1 -> Add_7ba88/2
  Alge_id_bus_2_38876/1 -> Product_2d9be/2
  Constant_376.991118430775_c52dd/1 -> Product_2bf68/1
  Product_2d9be/1 -> Add_7ba88/1
  State_vq_bus_2_b534c/1 -> Product_2bf68/2
  Add_7ba88/1 -> Blockout_d_vd_bus_2_81105/1

== system case1/AC_1/d_vd_bus_3_block ==
  note: d_vd_bus_3 in case1
      | $37699111.8430775\,\mathrm{id}_{\mathrm{bus},3}+376.991118430775\,\mathrm{vq}_{\mathrm{bus},3}$
      | Automatically generated on 2025-10-31 18:50:24 .
  Alge_id_bus_3_b8f2d : Inport
  State_vq_bus_3_2388c : Inport  Port=2
  Add_0ac10 : Sum
  Constant_376.991118430775_dda72 : Constant  Value=376.991118430775
  Constant_37699111.8430775_819e0 : Constant  Value=37699111.8430775
  Product_ac898 : Product
  Product_c40bb : Product
  Blockout_d_vd_bus_3_b64ce : Outport
  wires:
  Constant_37699111.8430775_819e0/1 -> Product_ac898/1
  Product_c40bb/1 -> Add_0ac10/2
  Alge_id_bus_3_b8f2d/1 -> Product_ac898/2
  Constant_376.991118430775_dda72/1 -> Product_c40bb/1
  Product_ac898/1 -> Add_0ac10/1
  State_vq_bus_3_2388c/1 -> Product_c40bb/2
  Add_0ac10/1 -> Blockout_d_vd_bus_3_b64ce/1

== system case1/AC_1/d_vd_bus_4_block ==
  note: d_vd_bus_4 in case1
      | $2257.43184689087\,\mathrm{id}_{\mathrm{bus},4}+376.991118430775\,\mathrm{vq}_{\mathrm{bus},4}$
      | Automatically generated on 2025-10-31 18:50:25 .
  Alge_id_bus_4_47562 : Inport
  State_vq_bus_4_5b78f : Inport  Port=2
  Add_9d53a : Sum
  Constant_2257.43184689087_f43c2 : Constant  Value=2257.43184689087
  Constant_376.991118430775_1194b : Constant  Value=376.991118430775
  Product_7382d : Product
  Product_a7a2a : Product
  Blockout_d_vd_bus_4_c0860 : Outport
  wires:
  Constant_2257.43184689087_f43c2/1 -> Product_a7a2a/1
  Product_7382d/1 -> Add_9d53a/2
  Alge_id_bus_4_47562/1 -> Product_a7a2a/2
  Constant_376.991118430775_1194b/1 -> Product_7382d/1
  Product_a7a2a/1 -> Add_9d53a/1
  State_vq_bus_4_5b78f/1 -> Product_7382d/2
  Add_9d53a/1 -> Blockout_d_vd_bus_4_c0860/1

== system case1/AC_1/d_vd_bus_5_block ==
  note: d_vd_bus_5 in case1
      | $1461.2058853906\,\mathrm{id}_{\mathrm{bus},5}+376.991118430775\,\mathrm{vq}_{\mathrm{bus},5}$
      | Automatically generated on 2025-10-31 18:50:27 .
  Alge_id_bus_5_af057 : Inport
  State_vq_bus_5_226eb : Inport  Port=2
  Add_9ff90 : Sum
  Constant_1461.2058853906_ae4ea : Constant  Value=1461.2058853906
  Constant_376.991118430775_6c2dd : Constant  Value=376.991118430775
  Product_4dce1 : Product
  Product_a1cef : Product
  Blockout_d_vd_bus_5_8fe13 : Outport
  wires:
  Constant_1461.2058853906_ae4ea/1 -> Product_4dce1/1
  Product_a1cef/1 -> Add_9ff90/2
  Alge_id_bus_5_af057/1 -> Product_4dce1/2
  Constant_376.991118430775_6c2dd/1 -> Product_a1cef/1
  Product_4dce1/1 -> Add_9ff90/1
  State_vq_bus_5_226eb/1 -> Product_a1cef/2
  Add_9ff90/1 -> Blockout_d_vd_bus_5_8fe13/1

== system case1/AC_1/d_vd_bus_6_block ==
  note: d_vd_bus_6 in case1
      | $1329.77466818616\,\mathrm{id}_{\mathrm{bus},6}+376.991118430775\,\mathrm{vq}_{\mathrm{bus},6}$
      | Automatically generated on 2025-10-31 18:50:29 .
  Alge_id_bus_6_1fc99 : Inport
  State_vq_bus_6_78a87 : Inport  Port=2
  Add_efe4b : Sum
  Constant_1329.77466818616_8e15f : Constant  Value=1329.77466818616
  Constant_376.991118430775_50fef : Constant  Value=376.991118430775
  Product_05a96 : Product
  Product_31365 : Product
  Blockout_d_vd_bus_6_d75a1 : Outport
  wires:
  Constant_1329.77466818616_8e15f/1 -> Product_05a96/1
  Product_31365/1 -> Add_efe4b/2
  Alge_id_bus_6_1fc99/1 -> Product_05a96/2
  Constant_376.991118430775_50fef/1 -> Product_31365/1
  Product_05a96/1 -> Add_efe4b/1
  State_vq_bus_6_78a87/1 -> Product_31365/2
  Add_efe4b/1 -> Blockout_d_vd_bus_6_d75a1/1

== system case1/AC_1/d_vd_bus_7_block ==
  note: d_vd_bus_7 in case1
      | $2106.09563369148\,\mathrm{id}_{\mathrm{bus},7}+376.991118430775\,\mathrm{vq}_{\mathrm{bus},7}$
      | Automatically generated on 2025-10-31 18:50:30 .
  Alge_id_bus_7_e5b9f : Inport
  State_vq_bus_7_885c9 : Inport  Port=2
  Add_770b5 : Sum
  Constant_2106.09563369148_3a13e : Constant  Value=2106.09563369148
  Constant_376.991118430775_e5908 : Constant  Value=376.991118430775
  Product_2cb43 : Product
  Product_b9c17 : Product
  Blockout_d_vd_bus_7_eeed9 : Outport
  wires:
  Constant_2106.09563369148_3a13e/1 -> Product_b9c17/1
  Product_2cb43/1 -> Add_770b5/2
  Alge_id_bus_7_e5b9f/1 -> Product_b9c17/2
  Constant_376.991118430775_e5908/1 -> Product_2cb43/1
  Product_b9c17/1 -> Add_770b5/1
  State_vq_bus_7_885c9/1 -> Product_2cb43/2
  Add_770b5/1 -> Blockout_d_vd_bus_7_eeed9/1

== system case1/AC_1/d_vd_bus_8_block ==
  note: d_vd_bus_8 in case1
      | $1657.10381727813\,\mathrm{id}_{\mathrm{bus},8}+376.991118430775\,\mathrm{vq}_{\mathrm{bus},8}$
      | Automatically generated on 2025-10-31 18:50:32 .
  Alge_id_bus_8_bb1f2 : Inport
  State_vq_bus_8_682c6 : Inport  Port=2
  Add_898e0 : Sum
  Constant_1657.10381727813_ce368 : Constant  Value=1657.10381727813
  Constant_376.991118430775_74c9a : Constant  Value=376.991118430775
  Product_de7d5 : Product
  Product_f12fb : Product
  Blockout_d_vd_bus_8_835b6 : Outport
  wires:
  Constant_1657.10381727813_ce368/1 -> Product_f12fb/1
  Product_de7d5/1 -> Add_898e0/2
  Alge_id_bus_8_bb1f2/1 -> Product_f12fb/2
  Constant_376.991118430775_74c9a/1 -> Product_de7d5/1
  Product_f12fb/1 -> Add_898e0/1
  State_vq_bus_8_682c6/1 -> Product_de7d5/2
  Add_898e0/1 -> Blockout_d_vd_bus_8_835b6/1

== system case1/AC_1/d_vd_bus_9_block ==
  note: d_vd_bus_9 in case1
      | $1564.27849971276\,\mathrm{id}_{\mathrm{bus},9}+376.991118430775\,\mathrm{vq}_{\mathrm{bus},9}$
      | Automatically generated on 2025-10-31 18:50:34 .
  Alge_id_bus_9_1ac5c : Inport
  State_vq_bus_9_a5e2a : Inport  Port=2
  Add_7b2ef : Sum
  Constant_1564.27849971276_240eb : Constant  Value=1564.27849971276
  Constant_376.991118430775_d2fb2 : Constant  Value=376.991118430775
  Product_89909 : Product
  Product_8b21f : Product
  Blockout_d_vd_bus_9_2d149 : Outport
  wires:
  Constant_1564.27849971276_240eb/1 -> Product_8b21f/1
  Product_89909/1 -> Add_7b2ef/2
  Alge_id_bus_9_1ac5c/1 -> Product_8b21f/2
  Constant_376.991118430775_d2fb2/1 -> Product_89909/1
  Product_8b21f/1 -> Add_7b2ef/1
  State_vq_bus_9_a5e2a/1 -> Product_89909/2
  Add_7b2ef/1 -> Blockout_d_vd_bus_9_2d149/1

== system case1/AC_1/d_vq_bus_1_block ==
  note: d_vq_bus_1 in case1
      | $37699111.8430775\,\mathrm{iq}_{\mathrm{bus},1}-376.991118430775\,\mathrm{vd}_{\mathrm{bus},1}$
      | Automatically generated on 2025-10-31 18:50:22 .
  Alge_iq_bus_1_aaaa9 : Inport
  State_vd_bus_1_fc5b3 : Inport  Port=2
  Constant_376.991118430775_83e8f : Constant  Value=376.991118430775
  Constant_37699111.8430775_998c3 : Constant  Value=37699111.8430775
  Product_0a28e : Product
  Product_58c27 : Product
  Subtract_6d166 : Sum  Inputs=+-
  Blockout_d_vq_bus_1_0a2d1 : Outport
  wires:
  Constant_37699111.8430775_998c3/1 -> Product_0a28e/1
  Constant_376.991118430775_83e8f/1 -> Product_58c27/1
  Alge_iq_bus_1_aaaa9/1 -> Product_0a28e/2
  State_vd_bus_1_fc5b3/1 -> Product_58c27/2
  Product_0a28e/1 -> Subtract_6d166/1
  Product_58c27/1 -> Subtract_6d166/2
  Subtract_6d166/1 -> Blockout_d_vq_bus_1_0a2d1/1

== system case1/AC_1/d_vq_bus_2_block ==
  note: d_vq_bus_2 in case1
      | $37699111.8430775\,\mathrm{iq}_{\mathrm{bus},2}-376.991118430775\,\mathrm{vd}_{\mathrm{bus},2}$
      | Automatically generated on 2025-10-31 18:50:23 .
  Alge_iq_bus_2_d5b4f : Inport
  State_vd_bus_2_40a78 : Inport  Port=2
  Constant_376.991118430775_8d6e9 : Constant  Value=376.991118430775
  Constant_37699111.8430775_aff44 : Constant  Value=37699111.8430775
  Product_4b3c2 : Product
  Product_cdb61 : Product
  Subtract_09273 : Sum  Inputs=+-
  Blockout_d_vq_bus_2_1031e : Outport
  wires:
  Constant_37699111.8430775_aff44/1 -> Product_cdb61/1
  Constant_376.991118430775_8d6e9/1 -> Product_4b3c2/1
  Alge_iq_bus_2_d5b4f/1 -> Product_cdb61/2
  State_vd_bus_2_40a78/1 -> Product_4b3c2/2
  Product_cdb61/1 -> Subtract_09273/1
  Product_4b3c2/1 -> Subtract_09273/2
  Subtract_09273/1 -> Blockout_d_vq_bus_2_1031e/1

== system case1/AC_1/d_vq_bus_3_block ==
  note: d_vq_bus_3 in case1
      | $37699111.8430775\,\mathrm{iq}_{\mathrm{bus},3}-376.991118430775\,\mathrm{vd}_{\mathrm{bus},3}$
      | Automatically generated on 2025-10-31 18:50:25 .
  Alge_iq_bus_3_939b5 : Inport
  State_vd_bus_3_ddba3 : Inport  Port=2
  Constant_376.991118430775_3a2c3 : Constant  Value=376.991118430775
  Constant_37699111.8430775_22606 : Constant  Value=37699111.8430775
  Product_5d4f9 : Product
  Product_b2e76 : Product
  Subtract_965ef : Sum  Inputs=+-
  Blockout_d_vq_bus_3_a043d : Outport
  wires:
  Constant_37699111.8430775_22606/1 -> Product_5d4f9/1
  Constant_376.991118430775_3a2c3/1 -> Product_b2e76/1
  Alge_iq_bus_3_939b5/1 -> Product_5d4f9/2
  State_vd_bus_3_ddba3/1 -> Product_b2e76/2
  Product_5d4f9/1 -> Subtract_965ef/1
  Product_b2e76/1 -> Subtract_965ef/2
  Subtract_965ef/1 -> Blockout_d_vq_bus_3_a043d/1

== system case1/AC_1/d_vq_bus_4_block ==
  note: d_vq_bus_4 in case1
      | $2257.43184689087\,\mathrm{iq}_{\mathrm{bus},4}-376.991118430775\,\mathrm{vd}_{\mathrm{bus},4}$
      | Automatically generated on 2025-10-31 18:50:26 .
  Alge_iq_bus_4_eaffa : Inport
  State_vd_bus_4_afc07 : Inport  Port=2
  Constant_2257.43184689087_407c9 : Constant  Value=2257.43184689087
  Constant_376.991118430775_819e0 : Constant  Value=376.991118430775
  Product_2a11b : Product
  Product_f88f5 : Product
  Subtract_67aa7 : Sum  Inputs=+-
  Blockout_d_vq_bus_4_e20db : Outport
  wires:
  Constant_2257.43184689087_407c9/1 -> Product_f88f5/1
  Constant_376.991118430775_819e0/1 -> Product_2a11b/1
  Alge_iq_bus_4_eaffa/1 -> Product_f88f5/2
  State_vd_bus_4_afc07/1 -> Product_2a11b/2
  Product_f88f5/1 -> Subtract_67aa7/1
  Product_2a11b/1 -> Subtract_67aa7/2
  Subtract_67aa7/1 -> Blockout_d_vq_bus_4_e20db/1

== system case1/AC_1/d_vq_bus_5_block ==
  note: d_vq_bus_5 in case1
      | $1461.2058853906\,\mathrm{iq}_{\mathrm{bus},5}-376.991118430775\,\mathrm{vd}_{\mathrm{bus},5}$
      | Automatically generated on 2025-10-31 18:50:28 .
  Alge_iq_bus_5_a9f44 : Inport
  State_vd_bus_5_1574f : Inport  Port=2
  Constant_1461.2058853906_65782 : Constant  Value=1461.2058853906
  Constant_376.991118430775_c2e13 : Constant  Value=376.991118430775
  Product_3518f : Product
  Product_68d4d : Product
  Subtract_a8645 : Sum  Inputs=+-
  Blockout_d_vq_bus_5_d5d5a : Outport
  wires:
  Constant_1461.2058853906_65782/1 -> Product_68d4d/1
  Constant_376.991118430775_c2e13/1 -> Product_3518f/1
  Alge_iq_bus_5_a9f44/1 -> Product_68d4d/2
  State_vd_bus_5_1574f/1 -> Product_3518f/2
  Product_68d4d/1 -> Subtract_a8645/1
  Product_3518f/1 -> Subtract_a8645/2
  Subtract_a8645/1 -> Blockout_d_vq_bus_5_d5d5a/1

== system case1/AC_1/d_vq_bus_6_block ==
  note: d_vq_bus_6 in case1
      | $1329.77466818616\,\mathrm{iq}_{\mathrm{bus},6}-376.991118430775\,\mathrm{vd}_{\mathrm{bus},6}$
      | Automatically generated on 2025-10-31 18:50:30 .
  Alge_iq_bus_6_2e2a2 : Inport
  State_vd_bus_6_e07dd : Inport  Port=2
  Constant_1329.77466818616_28ee0 : Constant  Value=1329.77466818616
  Constant_376.991118430775_2a869 : Constant  Value=376.991118430775
  Product_ce794 : Product
  Product_d7ad8 : Product
  Subtract_17aff : Sum  Inputs=+-
  Blockout_d_vq_bus_6_1e8a2 : Outport
  wires:
  Constant_1329.77466818616_28ee0/1 -> Product_d7ad8/1
  Constant_376.991118430775_2a869/1 -> Product_ce794/1
  Alge_iq_bus_6_2e2a2/1 -> Product_d7ad8/2
  State_vd_bus_6_e07dd/1 -> Product_ce794/2
  Product_d7ad8/1 -> Subtract_17aff/1
  Product_ce794/1 -> Subtract_17aff/2
  Subtract_17aff/1 -> Blockout_d_vq_bus_6_1e8a2/1
